simulink model "sampleModel158"  (R2021b)
settings: Solver=VariableStepAuto  StartTime=0.0  StopTime=10.0  RelTol=1e-3
undefined symbols (not defined in the file or in its folder): DiscIntNeverNeededParam, Newton, Raphson
libraries: simulink x9
settings Model: Creator=user  LastModifiedBy=user

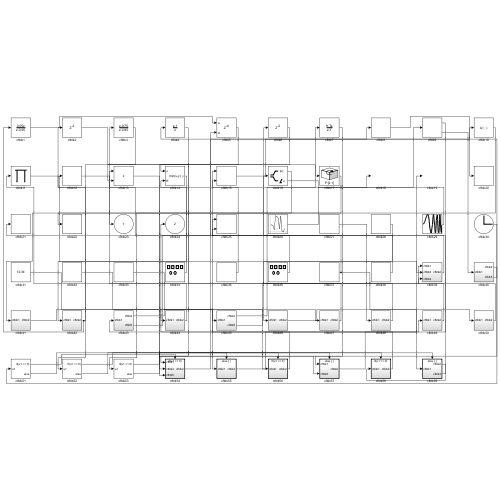
[thumbnail: Simulink's stored preview of the top-level diagram]
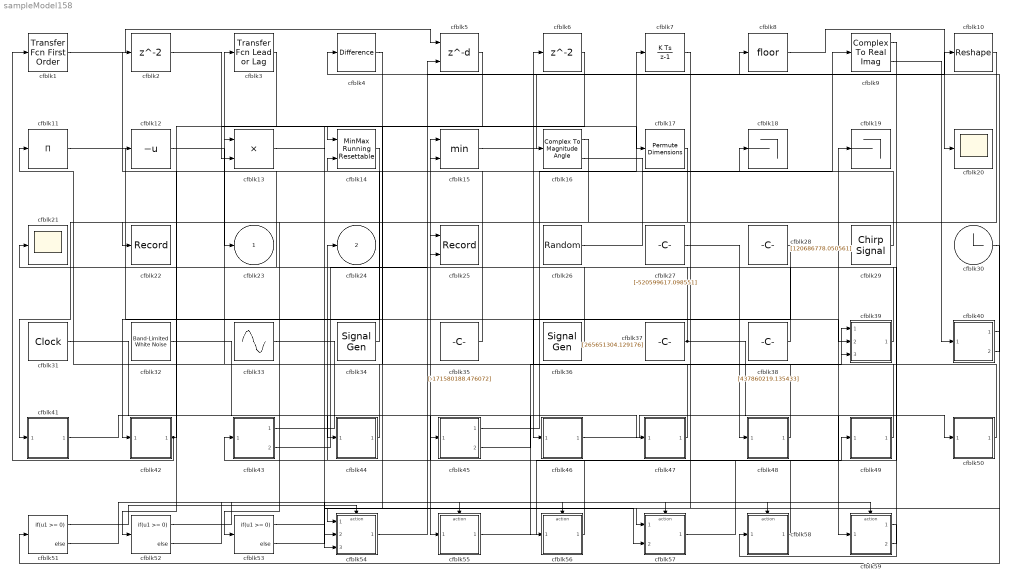
== system sampleModel158 ==
  cfblk1 : simulink/Discrete/Transfer Fcn First Order  PoleZ=0.95  ICPrevOutput=0.0  DoSatur=off
  cfblk10 : Reshape
  cfblk11 : Product  Inputs=*
  cfblk12 : UnaryMinus
  cfblk13 : Product  Inputs=**
  cfblk14 : simulink/Math Operations/MinMax Running Resettable  Function=min  vinit=0.0
  cfblk15 : MinMax  Inputs=2
  cfblk16 : ComplexToMagnitudeAngle
  cfblk17 : PermuteDimensions
  cfblk18 : Terminator
  cfblk19 : Terminator
  cfblk2 : Delay  SampleTime=1
  cfblk20 : Scope
  cfblk21 : Scope
  cfblk22 : Record  FileSettingsInternal="{\"entries\":[{\"content\":{\"excelSettings\":{\"content\":{},\"type\":\"Streamout.ExcelSettings\"}},\"type\":\"Streamout.FileSettingStorage\",\"uuid\":\"3d8ad447-dfcb-4988-be51-32d93d39a4ce\"}],\"packageUris\":[\"http://schema.mathworks.com/mf0/streamout_blocks/R2020a\"],\"version\":\"1.0\"}"  SignalsInternal="{\"entries\":[{\"content\":{\"signals\":[{\"content\":{\"blockPath\":[\"sampleModel158/cfblk22\"],\"channel\":[],\"dimensions\":[1],\"domain\":\"sampleModel158/cfblk22\",\"lineColor\":\"#fe330a\",\"plots\":[1],\"port\":1,\"sid\":[\"\"],\"signalID\":5944,\"signalName\":\"cfblk16:1\"},\"type\":\"RecordBlkView.Signal\",\"uuid\":\"ca8fd051-0cff-4379-907a-f7e4da9e0aee\"}]},\"type\":\"RecordBlkView.InputSignals\",\"uuid\":\"9773acb8-5fd8-49b9-9c29-46ffebf82336\"}],\"packageUris\":[\"http://schema.mathworks.com/mf0/streamout_blocks/R2020a\"],\"version\":\"1.0\"}"  VisualizationBindings="{\"sparklinesplugin\":{\"info\":[{\"bindingParametersList\":[],\"subplotID\":1}]}}"
  cfblk25 : Record  FileSettingsInternal="{\"entries\":[{\"content\":{\"excelSettings\":{\"content\":{},\"type\":\"Streamout.ExcelSettings\"}},\"type\":\"Streamout.FileSettingStorage\",\"uuid\":\"b112123a-a63b-48c0-bff8-cf90cd7201c5\"}],\"packageUris\":[\"http://schema.mathworks.com/mf0/streamout_blocks/R2020a\"],\"version\":\"1.0\"}"  Layout=[1 1]  SignalsInternal="{\"entries\":[{\"content\":{\"signals\":[{\"content\":{\"blockPath\":[\"sampleModel158/cfblk25\"],\"channel\":[],\"dimensions\":[1],\"domain\":\"sampleModel158/cfblk25\",\"lineColor\":\"#a2142f\",\"plots\":[1],\"port\":1,\"sid\":[\"\"],\"signalID\":5936,\"signalName\":\"cfblk39\"},\"type\":\"RecordBlkView.Signal\",\"uuid\":\"5cd1db8c-e79a-4b33-adbb-e0f995d5e017\"},{\"content\":{\"blockPath\":[\"sampleModel158/cfblk25\"],\"channel\":[],\"dimensions\":[1],\"domain\":\"sampleModel158/cfblk25\",\"lineColor\":\"#139fff\",\"plots\":[1],\"port\":2,\"sid\":[\"\"],\"signalID\":5940,\"signalName\":\"cfblk59:2\"},\"type\":\"RecordBlkView.Signal\",\"uuid\":\"ad50c800-6d33-4b1e-89c4-2949c0dbca13\"}]},\"type\":\"RecordBlkView.InputSignals\",\"uuid\":\"85afabe1-4bca-4619-85de-bb02d1445e9d\"}],\"packageUris\":[\"http://schema.mathworks.com/mf0/streamout_blocks/R2020a\"],\"version\":\"1.0\"}"  VisualizationBindings="{\"xyplotplugin\":{\"info\":[{\"series\":[{\"bindingParametersList\":[{\"parameter\":\"X-Axis\",\"signalID\":5936,\"signalName\":\"cfblk39\"},{\"parameter\":\"Y-Axis\",\"signalID\":5940,\"signalName\":\"cfblk59:2\"}],\"seriesID\":56823}],\"subplotID\":1}]}}"  CompatibilityTag=XY
  cfblk26 : RandomNumber  Mean=[-7084.640662]  Variance=[16040.532154]  Seed=[895292948.000000]  SampleTime=0.1
  cfblk27 : Constant  Value=[-520599617.098551]  SampleTime=1
  cfblk28 : Constant  Value=[120686778.050561]  SampleTime=1
  cfblk29 : simulink/Sources/Chirp Signal  f1=[-324034088.709702]  T=[-829366603.386133]  f2=[464887955.040006]
  cfblk3 : simulink/Discrete/Transfer Fcn Lead or Lag  PoleZ=0.95  ZeroZ=0.75  ICPrevOutput=0.0  ICPrevInput=0.0  DoSatur=off
      settings: SourceProductBaseCode=SL
  cfblk30 : Clock
  cfblk31 : DigitalClock
  cfblk32 : simulink/Sources/Band-Limited White Noise  Cov=[49427420.449006]  Ts=0.1  seed=[3394793048.000000]
  cfblk33 : Sin  Amplitude=[-120247284.265731]  Bias=[-651720609.055492]  SampleTime=0
  cfblk34 : SignalGenerator  WaveForm=sawtooth  Amplitude=[-101802727.928526]  Units=rad/sec
  cfblk35 : Constant  Value=[-171580188.476072]  SampleTime=1
  cfblk36 : SignalGenerator  Amplitude=[814683367.479868]
  cfblk37 : Constant  Value=[265651304.129176]  SampleTime=1
  cfblk38 : Constant  Value=[437860219.135433]  SampleTime=1
  cfblk39 : Subsystem
  cfblk4 : simulink/Discrete/Difference  ICPrevInput=0.0  OutMin=[]  OutMax=[]  OutDataTypeStr=Inherit: Inherit via back propagation  OutDataType=fixdt(1, 16)  OutScaling=2^-10  DoSatur=off
  cfblk40 : Subsystem
  cfblk41 : Subsystem
  cfblk42 : Subsystem
  cfblk43 : Subsystem
  cfblk44 : Subsystem
  cfblk45 : Subsystem
  cfblk46 : Subsystem
  cfblk47 : Subsystem
  cfblk48 : Subsystem
  cfblk49 : Subsystem
  cfblk5 : Delay  DelayLengthSource=Input port  SampleTime=1
      settings: InputPortMap=u0,p1
  cfblk50 : Subsystem
  cfblk51 : If  IfExpression=u1 >= 0  SampleTime=1
  cfblk52 : If  IfExpression=u1 >= 0  SampleTime=1
  cfblk53 : If  IfExpression=u1 >= 0  SampleTime=1
  cfblk54 : Subsystem  TreatAsAtomicUnit=on
  cfblk55 : Subsystem  TreatAsAtomicUnit=on
  cfblk56 : Subsystem  TreatAsAtomicUnit=on
  cfblk57 : Subsystem  TreatAsAtomicUnit=on
  cfblk58 : Subsystem  TreatAsAtomicUnit=on
  cfblk59 : Subsystem  TreatAsAtomicUnit=on
  cfblk6 : Delay  SampleTime=1
  cfblk7 : DiscreteIntegrator  ICPrevOutput=DiscIntNeverNeededParam  ICPrevScaledInput=DiscIntNeverNeededParam
  cfblk8 : Rounding
  cfblk9 : ComplexToRealImag
  cfblk23 : Outport
  cfblk24 : Outport  Port=2
  wires:
  cfblk14/1 -> cfblk42/1(cfblk1)
  cfblk48/1(cfblk2) -> cfblk14/1
  cfblk9/1 -> cfblk43/1(cfblk1)
  cfblk49/1(cfblk2) -> cfblk39/1(cfblk1)
  cfblk45/1(cfblk2) -> cfblk7/1
  cfblk28/1 -> cfblk46/1(cfblk1)
  cfblk37/1 -> cfblk21/1, cfblk59/1(cfblk1)
  cfblk33/1 -> cfblk55/1(cfblk1)
  cfblk1/1 -> cfblk5/1
  cfblk55/1(cfblk2) -> cfblk19/1
  cfblk4/1 -> cfblk54/1(cfblk1)
  cfblk46/1(cfblk2) -> cfblk50/1(cfblk1)
  cfblk27/1 -> cfblk48/1(cfblk1)
  cfblk26/1 -> cfblk9/1
  cfblk58/1(cfblk2) -> cfblk15/1
  cfblk47/1(cfblk2) -> cfblk3/1
  cfblk8/1 -> cfblk20/1
  cfblk43/1(cfblk2) -> cfblk47/1(cfblk1)
  cfblk59/1(cfblk2) -> cfblk58/1(cfblk1)
  cfblk42/1(cfblk2) -> cfblk1/1, cfblk12/1
  cfblk15/1 -> cfblk10/1
  cfblk11/1 -> cfblk39/2(cfblk3)
  cfblk12/1 -> cfblk23/1
  cfblk31/1 -> cfblk45/1(cfblk1)
  cfblk16/1 -> cfblk22/1
  cfblk2/1 -> cfblk17/1
  cfblk17/1 -> cfblk53/1
  cfblk38/1 -> cfblk13/1
  cfblk57/1(cfblk2) -> cfblk49/1(cfblk1)
  cfblk6/1 -> cfblk52/1
  cfblk56/1(cfblk2) -> cfblk24/1
  cfblk45/2(cfblk5) -> cfblk39/3(cfblk4)
  cfblk29/1 -> cfblk14/2
  cfblk54/1(cfblk2) -> cfblk8/1
  cfblk32/1 -> cfblk56/1(cfblk1)
  cfblk36/1 -> cfblk6/1
  cfblk16/2 -> cfblk18/1
  cfblk39/1(cfblk2) -> cfblk25/1
  cfblk10/1 -> cfblk41/1(cfblk1)
  cfblk50/1(cfblk2) -> cfblk16/1
  cfblk43/2(cfblk5) -> cfblk5/2
  cfblk9/2 -> cfblk40/1(cfblk1)
  cfblk35/1 -> cfblk15/2
  cfblk3/1 -> cfblk13/2
  cfblk41/1(cfblk2) -> cfblk44/1(cfblk1)
  cfblk30/1 -> cfblk51/1
  cfblk40/1(cfblk2) -> cfblk54/2(cfblk4)
  cfblk5/1 -> cfblk54/3(cfblk5)
  cfblk40/2(cfblk5) -> cfblk4/1
  cfblk7/1 -> cfblk57/1(cfblk1)
  cfblk44/1(cfblk2) -> cfblk11/1
  cfblk13/1 -> cfblk57/2(cfblk5)
  cfblk59/2(cfblk3) -> cfblk25/2
  cfblk34/1 -> cfblk2/1
  cfblk51/1 -> cfblk54/Action
  cfblk51/2 -> cfblk55/Action
  cfblk52/1 -> cfblk56/Action
  cfblk52/2 -> cfblk57/Action
  cfblk53/1 -> cfblk58/Action
  cfblk53/2 -> cfblk59/Action

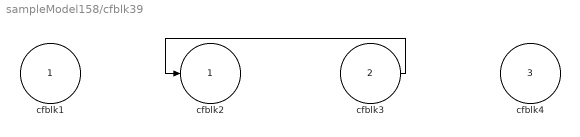
== system sampleModel158/cfblk39 ==
  cfblk1 : Inport
  cfblk3 : Inport  Port=2
  cfblk4 : Inport  Port=3
  cfblk2 : Outport
  wires:
  cfblk3/1 -> cfblk2/1

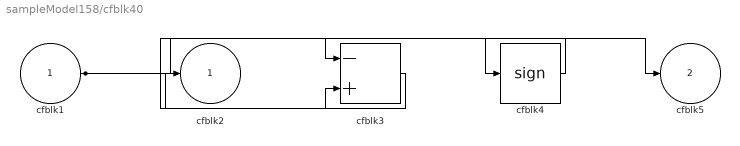
== system sampleModel158/cfblk40 ==
  cfblk1 : Inport
  cfblk3 : Sum  Inputs=-+
  cfblk4 : Signum
  cfblk2 : Outport
  cfblk5 : Outport  Port=2
  wires:
  cfblk1/1 -> cfblk5/1, cfblk4/1, cfblk3/2
  cfblk3/1 -> cfblk2/1
  cfblk4/1 -> cfblk3/1

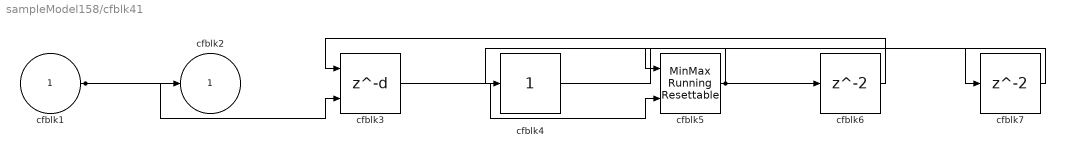
== system sampleModel158/cfblk41 ==
  cfblk1 : Inport
  cfblk3 : Delay  DelayLengthSource=Input port  SampleTime=1
      settings: InputPortMap=u0,p1
  cfblk4 : simulink/Math Operations/Slider Gain  gain=1  low=0  high=2
  cfblk5 : simulink/Math Operations/MinMax Running Resettable  Function=min  vinit=0.0
  cfblk6 : Delay  SampleTime=1
  cfblk7 : Delay  SampleTime=1
  cfblk2 : Outport
  wires:
  cfblk1/1 -> cfblk2/1, cfblk3/2
  cfblk5/1 -> cfblk4/1, cfblk6/1
  cfblk3/1 -> cfblk5/2
  cfblk6/1 -> cfblk3/1
  cfblk4/1 -> cfblk7/1
  cfblk7/1 -> cfblk5/1

== system sampleModel158/cfblk42 ==
  cfblk1 : Inport
  cfblk3 : DiscreteZeroPole  Poles=[0 0.5]  Gain=1
  cfblk2 : Outport
  wires:
  cfblk1/1 -> cfblk3/1
  cfblk3/1 -> cfblk2/1

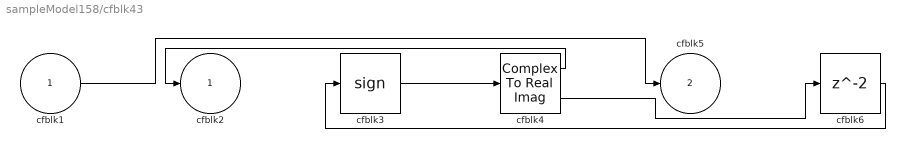
== system sampleModel158/cfblk43 ==
  cfblk1 : Inport
  cfblk3 : Signum
  cfblk4 : ComplexToRealImag
  cfblk6 : Delay  SampleTime=1
  cfblk2 : Outport
  cfblk5 : Outport  Port=2
  wires:
  cfblk3/1 -> cfblk4/1
  cfblk4/1 -> cfblk2/1
  cfblk1/1 -> cfblk5/1
  cfblk4/2 -> cfblk6/1
  cfblk6/1 -> cfblk3/1

== system sampleModel158/cfblk44 ==
  cfblk1 : Inport
  cfblk3 : Delay  DelayLengthSource=Input port  SampleTime=1
      settings: InputPortMap=u0,p1
  cfblk4 : DiscreteFir  SampleTime=1
  cfblk2 : Outport
  wires:
  cfblk3/1 -> cfblk2/1
  cfblk1/1 -> cfblk4/1
  cfblk4/1 -> cfblk3/1, cfblk3/2

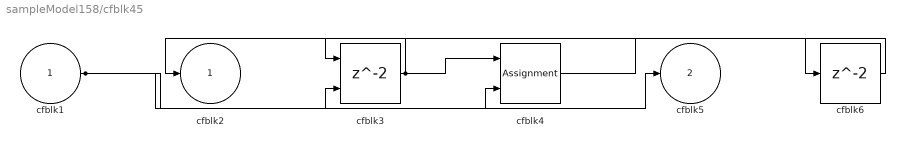
== system sampleModel158/cfblk45 ==
  cfblk1 : Inport
  cfblk3 : Delay  ShowEnablePort=on  SampleTime=1
      settings: InputPortMap=u0,e6
  cfblk4 : Assignment  DiagnosticForDimensions=Warning  IndexOptions=Index vector (dialog)  Indices=1  OutputSizes=1
  cfblk6 : Delay  SampleTime=1
  cfblk2 : Outport
  cfblk5 : Outport  Port=2
  wires:
  cfblk3/1 -> cfblk2/1, cfblk4/1
  cfblk1/1 -> cfblk5/1, cfblk3/2, cfblk4/2
  cfblk4/1 -> cfblk6/1
  cfblk6/1 -> cfblk3/1

== system sampleModel158/cfblk46 ==
  cfblk1 : Inport
  cfblk3 : Sqrt  Operator=rSqrt  AlgorithmType=Newton-Raphson  SaturateOnIntegerOverflow=on
  cfblk2 : Outport
  wires:
  cfblk1/1 -> cfblk3/1
  cfblk3/1 -> cfblk2/1

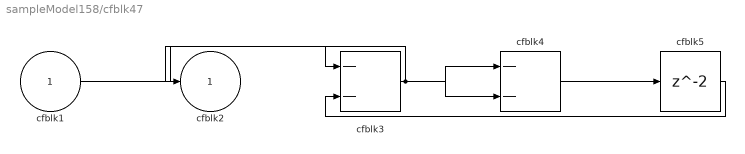
== system sampleModel158/cfblk47 ==
  cfblk1 : Inport
  cfblk3 : Sum  Inputs=--
  cfblk4 : Sum  Inputs=--
  cfblk5 : Delay  SampleTime=1
  cfblk2 : Outport
  wires:
  cfblk1/1 -> cfblk3/1
  cfblk3/1 -> cfblk4/1, cfblk2/1, cfblk4/2
  cfblk4/1 -> cfblk5/1
  cfblk5/1 -> cfblk3/2

== system sampleModel158/cfblk48 ==
  cfblk1 : Inport
  cfblk3 : Constant  Value=[-28610231.143134]  SampleTime=1
  cfblk2 : Outport
  wires:
  cfblk3/1 -> cfblk2/1

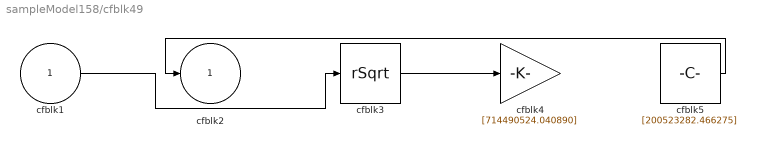
== system sampleModel158/cfblk49 ==
  cfblk1 : Inport
  cfblk3 : Sqrt  Operator=rSqrt  AlgorithmType=Newton-Raphson  SaturateOnIntegerOverflow=on
  cfblk4 : Gain  Gain=[714490524.040890]
  cfblk5 : Constant  Value=[200523282.466275]  SampleTime=1
  cfblk2 : Outport
  wires:
  cfblk5/1 -> cfblk2/1
  cfblk1/1 -> cfblk3/1
  cfblk3/1 -> cfblk4/1

== system sampleModel158/cfblk50 ==
  cfblk1 : Inport
  cfblk3 : Product  Inputs=**
  cfblk2 : Outport
  wires:
  cfblk1/1 -> cfblk3/1, cfblk3/2
  cfblk3/1 -> cfblk2/1

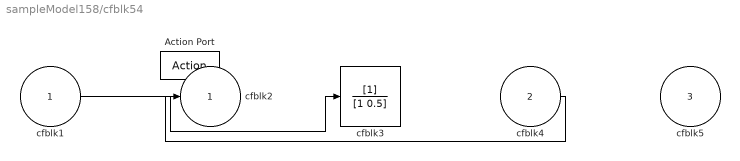
== system sampleModel158/cfblk54 ==
  cfblk1 : Inport
  cfblk4 : Inport  Port=2
  cfblk5 : Inport  Port=3
  Action Port : ActionPort  ActionPortLabel=if(u1 >= 0)
  cfblk3 : DiscreteFilter
  cfblk2 : Outport
  wires:
  cfblk1/1 -> cfblk3/1
  cfblk4/1 -> cfblk2/1

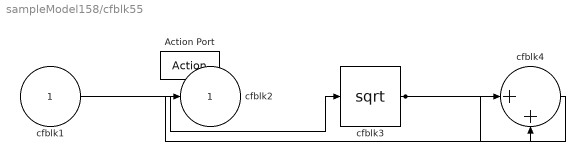
== system sampleModel158/cfblk55 ==
  cfblk1 : Inport
  Action Port : ActionPort  ActionPortLabel=else
  cfblk3 : Sqrt  SaturateOnIntegerOverflow=on
  cfblk4 : Sum  Inputs=|++
  cfblk2 : Outport
  wires:
  cfblk1/1 -> cfblk3/1
  cfblk3/1 -> cfblk4/1, cfblk4/2
  cfblk4/1 -> cfblk2/1

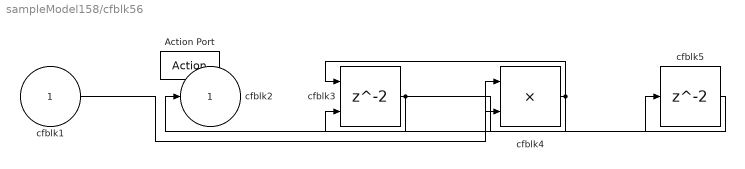
== system sampleModel158/cfblk56 ==
  cfblk1 : Inport
  Action Port : ActionPort  ActionPortLabel=if(u1 >= 0)
  cfblk3 : Delay  ShowEnablePort=on
      settings: InputPortMap=u0,e6
  cfblk4 : Product  Inputs=**
  cfblk5 : Delay
  cfblk2 : Outport
  wires:
  cfblk3/1 -> cfblk2/1, cfblk5/1
  cfblk4/1 -> cfblk3/1, cfblk3/2
  cfblk1/1 -> cfblk4/1
  cfblk5/1 -> cfblk4/2

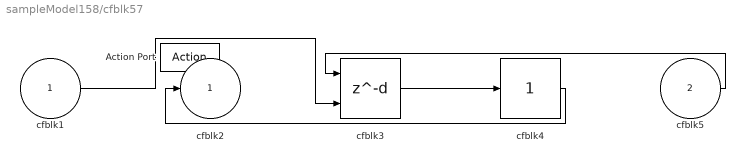
== system sampleModel158/cfblk57 ==
  cfblk1 : Inport
  cfblk5 : Inport  Port=2
  Action Port : ActionPort  ActionPortLabel=else
  cfblk3 : Delay  DelayLengthSource=Input port
      settings: InputPortMap=u0,p1
  cfblk4 : simulink/Math Operations/Slider Gain  gain=1  low=0  high=2
  cfblk2 : Outport
  wires:
  cfblk4/1 -> cfblk2/1
  cfblk3/1 -> cfblk4/1
  cfblk5/1 -> cfblk3/1
  cfblk1/1 -> cfblk3/2

== system sampleModel158/cfblk58 ==
  cfblk1 : Inport
  Action Port : ActionPort  ActionPortLabel=if(u1 >= 0)
  cfblk3 : ComplexToRealImag
  cfblk2 : Outport
  wires:
  cfblk3/1 -> cfblk2/1
  cfblk1/1 -> cfblk3/1

== system sampleModel158/cfblk59 ==
  cfblk1 : Inport
  Action Port : ActionPort  ActionPortLabel=else
  cfblk2 : Outport
  cfblk3 : Outport  Port=2
  wires:
  cfblk1/1 -> cfblk2/1, cfblk3/1
